simulink model "increment"  (Simulink 7.8)
settings: Solver=ode45  StartTime=0.0  StopTime=10.0  RelTol=1e-3
StopFcn:
  | incrementVars('increment')
settings Model: Creator=mkatz  LastModifiedBy=eric
settings OptimizationCC: InitFltsAndDblsToZero=on
settings DebuggingCC: SaveWithParameterizedLinksMsg=none  SignalResolutionControl=TryResolveAllWithWarning  MultiTaskDSMMsg=warning  MultiTaskCondExecSysMsg=none  FcnCallInpInsideContextMsg=Use local settings  StrictBusMsg=Warning
settings RTWCC: IncludeERTFirstTime=on
settings GRTTargetCC: TargetFcnLib=ansi_tfl_tmw.mat

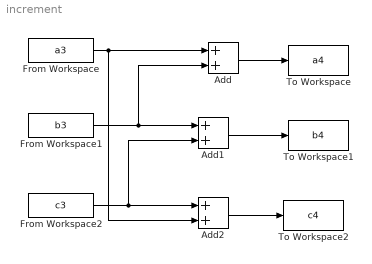
== system increment ==
  Add : Sum
  Add1 : Sum
  Add2 : Sum
  From Workspace : FromWorkspace  VariableName=a3  SampleTime=0
  From Workspace1 : FromWorkspace  VariableName=b3  SampleTime=0
  From Workspace2 : FromWorkspace  VariableName=c3  SampleTime=0
  To Workspace : ToWorkspace  VariableName=a4  SampleTime=-1  SaveFormat=Structure
  To Workspace1 : ToWorkspace  VariableName=b4  SampleTime=-1  SaveFormat=Structure
  To Workspace2 : ToWorkspace  VariableName=c4  SampleTime=-1  SaveFormat=Structure
  wires:
  From Workspace/1 -> Add/1, Add2/2
  From Workspace1/1 -> Add1/1, Add/2
  From Workspace2/1 -> Add1/2, Add2/1
  Add/1 -> To Workspace/1
  Add1/1 -> To Workspace1/1
  Add2/1 -> To Workspace2/1
